simulink library "ClairvauxLibrary"  (R2020b)
settings: Solver=VariableStepAuto  StartTime=0.0  StopTime=10.0  RelTol=1e-3
undefined symbols (not defined in the file): OutMax, OutMin, Ts, w0
libraries: $bdroot x4, simulink x2, sharedtransform x2
(part 1 of 2)
settings Model: Creator=mujim  LastModifiedBy=mujim

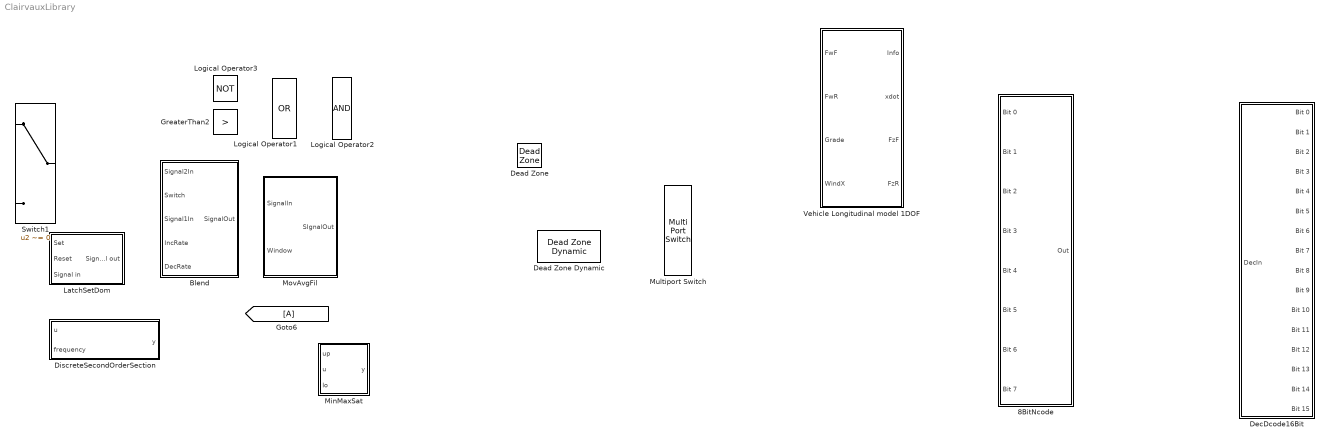
== system ClairvauxLibrary ==
  8BitNcode : Subsystem
  Blend : Subsystem
  Dead Zone : DeadZone  SaturateOnIntegerOverflow=on
  Dead Zone Dynamic : simulink/Discontinuities/Dead Zone Dynamic
      settings: SourceProductBaseCode=SL
  DecDcode16Bit : Subsystem
  DiscreteSecondOrderSection : Subsystem  mask(DiscreteSecondOrderSection){zeta=sin(1*pi/4), Ts=Ts, w0=w0}
      mask prompts: zeta "Damping ratio"; Ts "Sample time Ts"; w0 "Pre-warping frequency w0"
      mask help:
      | Implements the Tustin discretization of the second-order lowpass filter
      |
      |                          w^2
      | F(s) = ---------------------------------------
      |            s^2 + 2 * zeta * w * s + w^2
      |
      | where zeta is the damping ratio and w is the cutoff frequency value fed to the "frequency" port. The discrete transfer function is obtained by Tustin transformation with pre-warping at the frequency w0. The default value w0=0 corresponds to the usual bilinear transformation:
      |
      | s = 2/Ts (z-1)/(z+1).
      mask init:
      | if w0>0
      |    tau = tan(w0*Ts/2)/w0;
      | else
      |    tau = Ts/2;
      | end
      mask Display:
      | text(0.4,0.5,'DSOS');
      | port_label('input', 1, 'SigIn');
      | port_label('output', 1, 'SigOut');
      | port_label('input', 2, 'freq');
  GreaterThan2 : RelationalOperator  Operator=>  OutDataTypeStr=boolean  RndMeth=Zero
  LatchSetDom : Subsystem
  Logical Operator1 : Logic  Operator=OR  AllPortsSameDT=off  OutDataTypeStr=boolean
  Logical Operator2 : Logic  AllPortsSameDT=off  OutDataTypeStr=boolean
  Logical Operator3 : Logic  Operator=NOT  OutDataTypeStr=boolean
  MinMaxSat : Subsystem
  MovAvgFil : Subsystem
  Multiport Switch : MultiPortSwitch  Inputs=2  DataPortForDefault=Additional data port  DiagnosticForDefault=None  RndMeth=Zero
  Switch1 : Switch  Criteria=u2 ~= 0  OutDataTypeStr=double  RndMeth=Zero
  Vehicle Longitudinal model 1DOF : Subsystem  mask(Vehicle Longitudinal model 1DOF){NF=0, NR=0, m=0, a=0, b=0, h=0, Cd=0, Cl=0, Cpm=0, Af=0, x_o=0, xdot_o=0, Pabs=0, T=0, g=0}
      mask prompts: NF "Number of wheels on front axle, NF [-]"; NR "Number of wheels on rear axle, NR [-]"; m "Mass, m [Kg]"; a "Horizontal distance from CG to front axle, a [m]"; b "Horizontal distance from CG to rear axle, b [m]"; h "CG height above axles, h [m]"; Cd "Drag coefficient, Cd [-]"; Cl "Lift coefficient, Cl [-]"; Cpm "Pitch drag moment coeffiecient, Cpm [-]"; Af "Frontal Area, Af [m^2]"; x_o "Initial position, x_o [m]"; xdot_o "Initial velocity, xdot_o [m/s]"; Pabs "Absolute Pressure, Pabs [Pa]"; T "Air Temp, T [K]"; g "Gravitational acceleration, g [m/s^2]"
      mask DialogControl Container3 Prompt: Parameters
      mask DialogControl Container4 Prompt: Vehicle Paramters
      mask DialogControl Container11 Prompt: Environmental Parameters

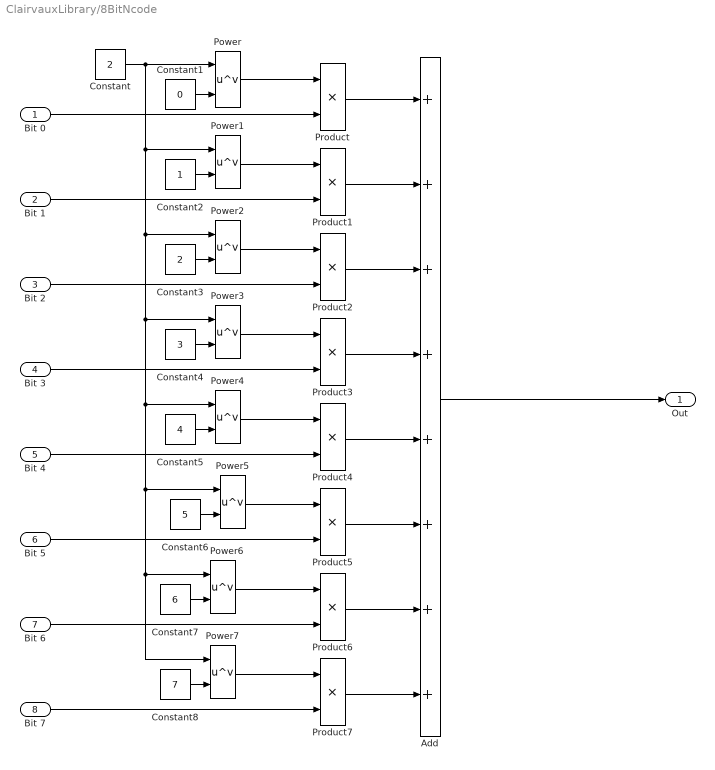
== system ClairvauxLibrary/8BitNcode ==
  Bit 0 : Inport
  Bit 1 : Inport  Port=2
  Bit 2 : Inport  Port=3
  Bit 3 : Inport  Port=4
  Bit 4 : Inport  Port=5
  Bit 5 : Inport  Port=6
  Bit 6 : Inport  Port=7
  Bit 7 : Inport  Port=8
  Add : Sum  Inputs=++++++++
  Constant : Constant  Value=2
  Constant1 : Constant  Value=0
  Constant2 : Constant
  Constant3 : Constant  Value=2
  Constant4 : Constant  Value=3
  Constant5 : Constant  Value=4
  Constant6 : Constant  Value=5
  Constant7 : Constant  Value=6
  Constant8 : Constant  Value=7
  Power{,1..7} (8 alike) : Math  Operator=pow  SaturateOnIntegerOverflow=on
  Product{,1..7} (8 alike) : Product
  Out : Outport
  wires:
  Bit 0/1 -> Product/2
  Constant/1 -> Power/1, Power1/1, Power2/1, Power3/1, Power7/1, Power6/1, Power5/1, Power4/1
  Power/1 -> Product/1
  Add/1 -> Out/1
  Constant1/1 -> Power/2
  Constant2/1 -> Power1/2
  Constant3/1 -> Power2/2
  Constant4/1 -> Power3/2
  Constant5/1 -> Power4/2
  Constant6/1 -> Power5/2
  Constant7/1 -> Power6/2
  Constant8/1 -> Power7/2
  Product/1 -> Add/1
  Product1/1 -> Add/2
  Product2/1 -> Add/3
  Product3/1 -> Add/4
  Product4/1 -> Add/5
  Product5/1 -> Add/6
  Product6/1 -> Add/7
  Product7/1 -> Add/8
  Power1/1 -> Product1/1
  Power2/1 -> Product2/1
  Power3/1 -> Product3/1
  Power4/1 -> Product4/1
  Power5/1 -> Product5/1
  Power6/1 -> Product6/1
  Power7/1 -> Product7/1
  Bit 1/1 -> Product1/2
  Bit 2/1 -> Product2/2
  Bit 3/1 -> Product3/2
  Bit 4/1 -> Product4/2
  Bit 5/1 -> Product5/2
  Bit 6/1 -> Product6/2
  Bit 7/1 -> Product7/2

== system ClairvauxLibrary/Blend ==
  note: Blend between 2 signals with a defined rate of rise and fall
      | Switch input:
      | 0 = Signal1
      | 1 = Signal2
  Signal2In : Inport
  Switch : Inport  Port=2
  Signal1In : Inport  Port=3
  IncRate : Inport  Port=4
  DecRate : Inport  Port=5
  Rate Limiter Dynamic : simulink/Discontinuities/Rate Limiter Dynamic
  Switch3 : $bdroot/Switch1  Criteria=u2 ~= 0  Threshold=0  OutMin=[]  OutMax=[]  OutDataTypeStr=double  RndMeth=Zero  SampleTime=-1  AllowDiffInputSizes=off
  SignalOut : Outport
  wires:
  Signal2In/1 -> Switch3/1
  Switch3/1 -> Rate Limiter Dynamic/2
  Rate Limiter Dynamic/1 -> SignalOut/1
  Signal1In/1 -> Switch3/3
  DecRate/1 -> Rate Limiter Dynamic/3
  Switch/1 -> Switch3/2
  IncRate/1 -> Rate Limiter Dynamic/1

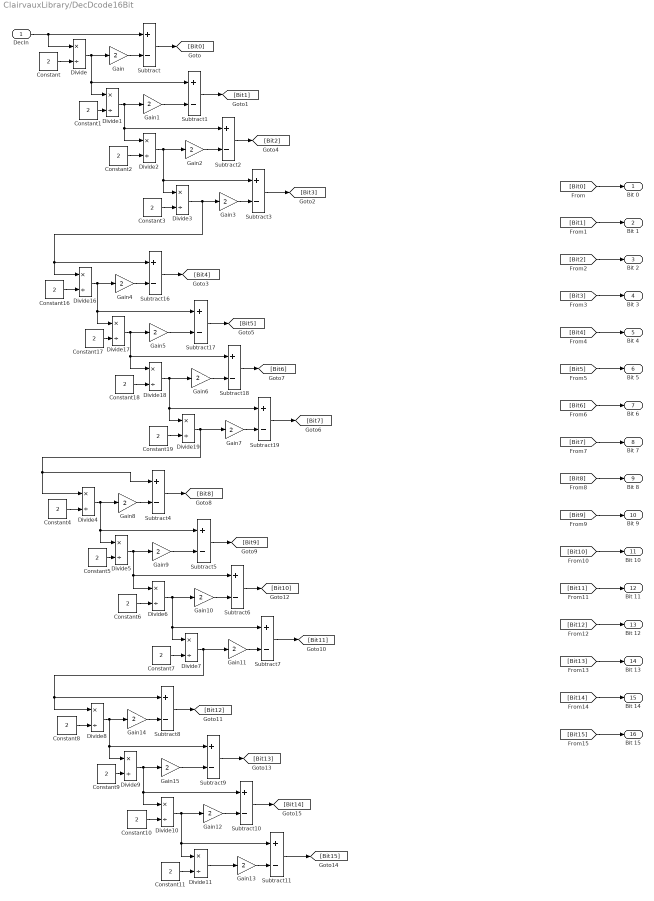
== system ClairvauxLibrary/DecDcode16Bit ==
  DecIn : Inport
  Constant{,1..11,16..19} (16 alike) : Constant  Value=2
  Divide{,1..11,16..19} (16 alike) : Product  Inputs=*/  OutDataTypeStr=fixdt('int16', 'DataTypeOverride', 'Off')
  Gain{,1..15} (16 alike) : Gain  Gain=2
  Subtract{,1..11,16..19} (16 alike) : Sum  Inputs=+-
  Bit 0 : Outport
  Bit 1 : Outport  Port=2
  Bit 2 : Outport  Port=3
  Bit 3 : Outport  Port=4
  Bit 4 : Outport  Port=5
  Bit 5 : Outport  Port=6
  Bit 6 : Outport  Port=7
  Bit 7 : Outport  Port=8
  Bit 8 : Outport  Port=9
  Bit 9 : Outport  Port=10
  Bit 10 : Outport  Port=11
  Bit 11 : Outport  Port=12
  Bit 12 : Outport  Port=13
  Bit 13 : Outport  Port=14
  Bit 14 : Outport  Port=15
  Bit 15 : Outport  Port=16
  wires:
  DecIn/1 -> Subtract/1, Divide/1
  Constant/1 -> Divide/2
  Divide/1 -> Divide1/1, Subtract1/1, Gain/1
  Divide1/1 -> Divide2/1, Subtract2/1, Gain1/1
  Constant1/1 -> Divide1/2
  Subtract/1 -> [Bit0]
  Constant2/1 -> Divide2/2
  Divide2/1 -> Divide3/1, Subtract3/1, Gain2/1
  [Bit0] -> Bit 0/1
  Subtract1/1 -> [Bit1]
  [Bit1] -> Bit 1/1
  Subtract3/1 -> [Bit3]
  Constant3/1 -> Divide3/2
  Subtract2/1 -> [Bit2]
  [Bit2] -> Bit 2/1
  [Bit3] -> Bit 3/1
  [Bit4] -> Bit 4/1
  [Bit5] -> Bit 5/1
  [Bit6] -> Bit 6/1
  [Bit7] -> Bit 7/1
  [Bit15] -> Bit 15/1
  [Bit14] -> Bit 14/1
  [Bit13] -> Bit 13/1
  [Bit12] -> Bit 12/1
  [Bit11] -> Bit 11/1
  [Bit10] -> Bit 10/1
  [Bit9] -> Bit 9/1
  [Bit8] -> Bit 8/1
  Gain/1 -> Subtract/2
  Gain1/1 -> Subtract1/2
  Gain2/1 -> Subtract2/2
  Gain3/1 -> Subtract3/2
  Gain7/1 -> Subtract19/2
  Gain6/1 -> Subtract18/2
  Gain5/1 -> Subtract17/2
  Gain4/1 -> Subtract16/2
  Divide19/1 -> Gain7/1, Subtract4/1, Divide4/1
  Subtract18/1 -> [Bit6]
  Constant19/1 -> Divide19/2
  Subtract19/1 -> [Bit7]
  Subtract17/1 -> [Bit5]
  Divide18/1 -> Gain6/1, Subtract19/1, Divide19/1
  Constant18/1 -> Divide18/2
  Subtract16/1 -> [Bit4]
  Constant17/1 -> Divide17/2
  Divide17/1 -> Gain5/1, Subtract18/1, Divide18/1
  Divide16/1 -> Gain4/1, Subtract17/1, Divide17/1
  Constant16/1 -> Divide16/2
  Divide3/1 -> Subtract16/1, Divide16/1, Gain3/1
  Constant4/1 -> Divide4/2
  Divide4/1 -> Divide5/1, Subtract5/1, Gain8/1
  Divide5/1 -> Divide6/1, Subtract6/1, Gain9/1
  Constant5/1 -> Divide5/2
  Subtract4/1 -> [Bit8]
  Constant6/1 -> Divide6/2
  Divide6/1 -> Divide7/1, Subtract7/1, Gain10/1
  Subtract5/1 -> [Bit9]
  Subtract7/1 -> [Bit11]
  Constant7/1 -> Divide7/2
  Subtract6/1 -> [Bit10]
  Divide7/1 -> Subtract8/1, Divide8/1, Gain11/1
  Gain8/1 -> Subtract4/2
  Gain9/1 -> Subtract5/2
  Gain10/1 -> Subtract6/2
  Gain11/1 -> Subtract7/2
  Gain13/1 -> Subtract11/2
  Gain12/1 -> Subtract10/2
  Gain15/1 -> Subtract9/2
  Gain14/1 -> Subtract8/2
  Divide11/1 -> Gain13/1
  Subtract10/1 -> [Bit14]
  Constant11/1 -> Divide11/2
  Subtract11/1 -> [Bit15]
  Subtract9/1 -> [Bit13]
  Divide10/1 -> Gain12/1, Subtract11/1, Divide11/1
  Constant10/1 -> Divide10/2
  Subtract8/1 -> [Bit12]
  Constant9/1 -> Divide9/2
  Divide9/1 -> Gain15/1, Subtract10/1, Divide10/1
  Divide8/1 -> Gain14/1, Subtract9/1, Divide9/1
  Constant8/1 -> Divide8/2

== system ClairvauxLibrary/DiscreteSecondOrderSection ==
  u : Inport
  frequency : Inport  Port=2
  Constant : Constant  Value=zeta
  Constant1 : Constant  Value=tau
  Gain1 : Gain  Gain=2
  MATLAB Function : MATLAB Function  Tag=#GainSurfaceTarget_  TreatAsAtomicUnit=on
  Product1 : Product
  Product2 : Product
  Product5 : Product
  Sum : Sum  Inputs=|++
  Sum1 : Sum  Inputs=++|
  Sum2 : Sum  Inputs=+|+
  Sum3 : Sum  Inputs=+|-
  Unit Delay1 : UnitDelay  SampleTime=Ts  HasFrameUpgradeWarning=on
  Unit Delay2 : UnitDelay  SampleTime=Ts  HasFrameUpgradeWarning=on
  y : Outport  VectorParamsAs1DForOutWhenUnconnected=off
  wires:
  Unit Delay1/1 -> Sum/2
  MATLAB Function/3(c) -> Product2/2
  MATLAB Function/2(b) -> Product5/2
  Product2/1 -> Sum3/2
  Constant1/1 -> MATLAB Function/3(tau)
  MATLAB Function/1(a) -> Product1/2
  frequency/1 -> MATLAB Function/1(w)
  Sum1/1 -> Unit Delay1/1
  Sum3/1 -> Unit Delay2/1
  Sum2/1 -> Gain1/1
  Constant/1 -> MATLAB Function/2(zeta)
  Product1/1 -> y/1
  u/1 -> Sum3/1, Sum2/1, Sum/1
  Unit Delay2/1 -> Sum1/2
  Sum/1 -> Product1/1, Product5/1, Product2/1
  Product5/1 -> Sum2/2
  Gain1/1 -> Sum1/1

== system ClairvauxLibrary/LatchSetDom ==
  Set : Inport
  Reset : Inport  Port=2
  Signal in : Inport  Port=3
  Signal out : Outport

== system ClairvauxLibrary/MinMaxSat ==
  up : Inport
  u : Inport  Port=2
  lo : Inport  Port=3
  LowerRelop1 : RelationalOperator  DisableCoverage=on  Operator=>  OutDataTypeStr=boolean  RndMeth=Nearest
  Switch : Switch  Criteria=u2 ~= 0  OutDataTypeStr=Inherit: Inherit via back propagation  ZeroCross=off
  Switch2 : Switch  Criteria=u2 ~= 0  OutMin=OutMin  OutMax=OutMax  OutDataTypeStr=Inherit: Inherit via back propagation  ZeroCross=off
  UpperRelop : RelationalOperator  DisableCoverage=on  Operator=<  OutDataTypeStr=boolean  RndMeth=Nearest
  y : Outport  OutMin=OutMin  OutMax=OutMax
  wires:
  Switch/1 -> Switch2/3
  LowerRelop1/1 -> Switch2/2
  UpperRelop/1 -> Switch/2
  Switch2/1 -> y/1
  u/1 -> LowerRelop1/1, Switch/3, UpperRelop/1
  up/1 -> Switch2/1, LowerRelop1/2
  lo/1 -> Switch/1, UpperRelop/2

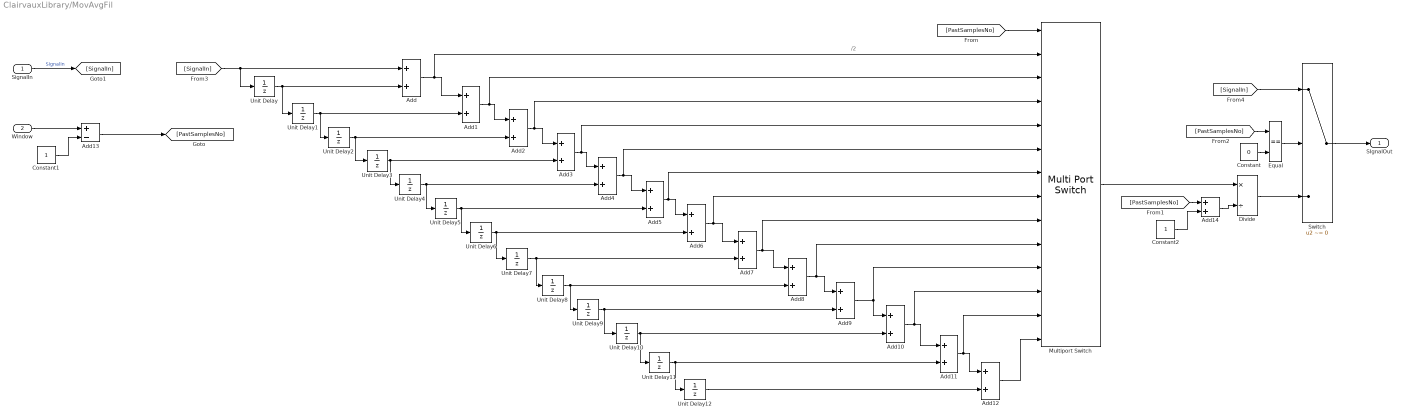
== system ClairvauxLibrary/MovAvgFil ==
  note: /2
  SignalIn : Inport
  Window : Inport  Port=2
  Add{,1..12,14} (14 alike) : Sum
  Add13 : Sum  Inputs=+-
  Constant : Constant  Value=0
  Constant1 : Constant
  Constant2 : Constant
  Divide : Product  Inputs=*/
  Equal : RelationalOperator  Operator===  OutDataTypeStr=boolean  RndMeth=Simplest
  Multiport Switch : MultiPortSwitch  Inputs=13
  Switch : Switch  Criteria=u2 ~= 0  RndMeth=Zero
  Unit Delay{,1..12} (13 alike) : UnitDelay  SampleTime=-1  HasFrameUpgradeWarning=on
  SIgnalOut : Outport
  wires:
  Divide/1 -> Switch/3
  [SignalIn] -> Switch/1
  Switch/1 -> SIgnalOut/1
  Equal/1 -> Switch/2
  [SignalIn] -> Unit Delay/1, Add/1
  Constant/1 -> Equal/2
  [PastSamplesNo] -> Equal/1
  [PastSamplesNo] -> Multiport Switch/1
  Multiport Switch/1 -> Divide/1
  Add12/1 -> Multiport Switch/14
  Add11/1 -> Multiport Switch/13, Add12/1
  Add10/1 -> Multiport Switch/12, Add11/1
  Unit Delay11/1 -> Unit Delay12/1, Add11/2
  Add9/1 -> Add10/1, Multiport Switch/11
  Add8/1 -> Multiport Switch/10, Add9/1
  Add7/1 -> Multiport Switch/9, Add8/1
  Add6/1 -> Multiport Switch/8, Add7/1
  Add5/1 -> Multiport Switch/7, Add6/1
  Add4/1 -> Multiport Switch/6, Add5/1
  Add3/1 -> Multiport Switch/5, Add4/1
  Add2/1 -> Multiport Switch/4, Add3/1
  Add1/1 -> Multiport Switch/3, Add2/1
  Add/1 -> Multiport Switch/2, Add1/1
  Unit Delay4/1 -> Unit Delay5/1, Add4/2
  Unit Delay2/1 -> Unit Delay3/1, Add2/2
  Unit Delay7/1 -> Add7/2, Unit Delay8/1
  Unit Delay8/1 -> Unit Delay9/1, Add8/2
  Unit Delay3/1 -> Unit Delay4/1, Add3/2
  Unit Delay12/1 -> Add12/2
  Unit Delay6/1 -> Add6/2, Unit Delay7/1
  SignalIn/1 -> [SignalIn]  "SignalIn"
  Unit Delay10/1 -> Unit Delay11/1, Add10/2
  Unit Delay1/1 -> Unit Delay2/1, Add1/2
  Unit Delay/1 -> Unit Delay1/1, Add/2
  Unit Delay9/1 -> Unit Delay10/1, Add9/2
  Unit Delay5/1 -> Add5/2, Unit Delay6/1
  Add13/1 -> [PastSamplesNo]
  Window/1 -> Add13/1
  Constant1/1 -> Add13/2
  Constant2/1 -> Add14/2
  [PastSamplesNo] -> Add14/1
  Add14/1 -> Divide/2

== system ClairvauxLibrary/Vehicle Longitudinal model 1DOF ==
  FwF : Inport
  FwR : Inport  Port=2
  Grade : Inport  Port=3
  WindX : Inport  Port=4
  AirTempConstant : Constant  Value=T
  FExtConstant : Constant  Value=[0,0,0]
  MExtConstant : Constant  Value=[0,0,0]
  Subsystem : Subsystem
  Info : Outport  VectorParamsAs1DForOutWhenUnconnected=off
  xdot : Outport  Port=2  PortDimensions=1  VectorParamsAs1DForOutWhenUnconnected=off
  FzF : Outport  Port=3  PortDimensions=1  VectorParamsAs1DForOutWhenUnconnected=off
  FzR : Outport  Port=4  PortDimensions=1  VectorParamsAs1DForOutWhenUnconnected=off
  wires:
  Subsystem/4(FzR) -> FzR/1
  FwF/1 -> Subsystem/1(FwF)
  FwR/1 -> Subsystem/2(FwR)
  Subsystem/1(Info) -> Info/1
  AirTempConstant/1 -> Subsystem/7(Temp)
  WindX/1 -> Subsystem/4(wind)
  MExtConstant/1 -> Subsystem/6(MExt)
  Subsystem/3(FzF) -> FzF/1
  FExtConstant/1 -> Subsystem/5(FExt)
  Grade/1 -> Subsystem/3(Grade)
  Subsystem/2(xdot) -> xdot/1

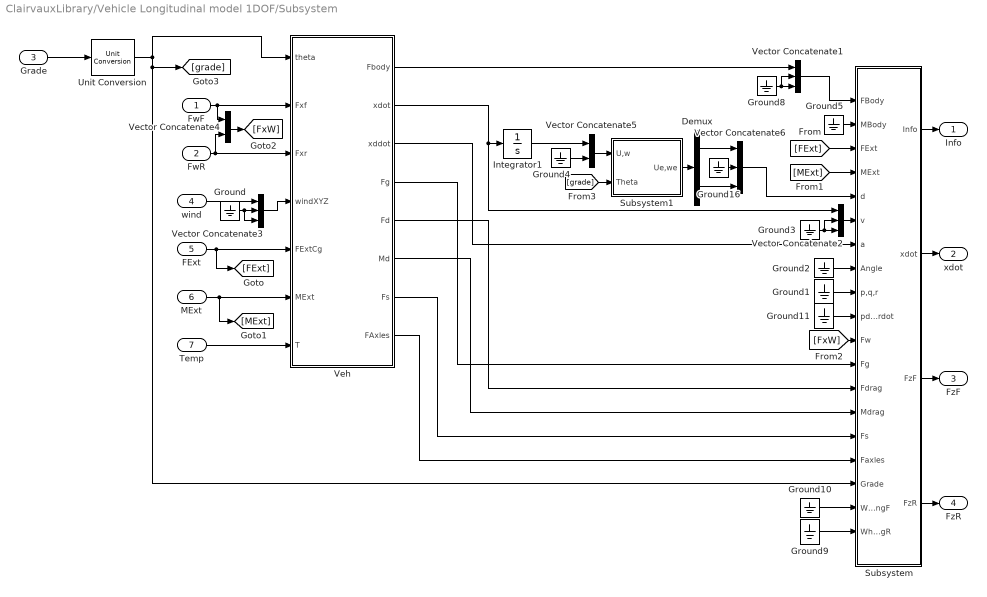
== system ClairvauxLibrary/Vehicle Longitudinal model 1DOF/Subsystem ==
  FwF : Inport  Unit=N
  FwR : Inport  Port=2  Unit=N
  Grade : Inport  Port=3  Unit=deg
  wind : Inport  Port=4  Unit=m/s
  FExt : Inport  Port=5  Unit=N
  MExt : Inport  Port=6  Unit=N*m
  Temp : Inport  Port=7  OutMin=eps  Unit=K
  Demux : Demux  Outputs=2
  Ground{,1..5,8..11,16} (11 alike) : Ground
  Integrator1 : Integrator  InitialCondition=x_o
  Subsystem : Subsystem
  Subsystem1 : Subsystem
  Unit Conversion : UnitConversion
  Vector Concatenate{1..3,6} (4 alike) : Concatenate  NumInputs=3
  Vector Concatenate4 : Concatenate
  Vector Concatenate5 : Concatenate
  Veh : Subsystem
  Info : Outport  VectorParamsAs1DForOutWhenUnconnected=off
  xdot : Outport  Port=2  Unit=m/s  VectorParamsAs1DForOutWhenUnconnected=off
  FzF : Outport  Port=3  Unit=N  VectorParamsAs1DForOutWhenUnconnected=off
  FzR : Outport  Port=4  Unit=N  VectorParamsAs1DForOutWhenUnconnected=off
  wires:
  MExt/1 -> Veh/6(MExt), [MExt]
  [MExt] -> Subsystem/4(MExt)
  Veh/7(Fs) -> Subsystem/15(Fs)
  Ground9/1 -> Subsystem/19(WhlAngR)
  Vector Concatenate5/1 -> Subsystem1/1(U,w)
  Ground4/1 -> Vector Concatenate5/2
  Ground16/1 -> Vector Concatenate6/2
  Veh/4(Fg) -> Subsystem/12(Fg)
  Demux/1 -> Vector Concatenate6/1
  Subsystem1/1(Ue,we) -> Demux/1
  Vector Concatenate3/1 -> Veh/4(windXYZ)
  Veh/5(Fd) -> Subsystem/13(Fdrag)
  Unit Conversion/1 -> Veh/1(theta), Subsystem/17(Grade), [grade]
  Ground5/1 -> Subsystem/2(MBody)
  [FxW] -> Subsystem/11(Fw)
  Ground11/1 -> Subsystem/10(pdot,qdot,rdot)
  Vector Concatenate2/1 -> Subsystem/6(v)
  Veh/3(xddot) -> Subsystem/7(a)
  Veh/6(Md) -> Subsystem/14(Mdrag)
  Demux/2 -> Vector Concatenate6/3
  FwF/1 -> Veh/2(Fxf), Vector Concatenate4/1
  Ground1/1 -> Subsystem/9(p,q,r)
  Subsystem/1(Info) -> Info/1
  Ground10/1 -> Subsystem/18(WhlAngF)
  FwR/1 -> Veh/3(Fxr), Vector Concatenate4/2
  Subsystem/4(FzR) -> FzR/1
  Vector Concatenate4/1 -> [FxW]
  Veh/8(FAxles) -> Subsystem/16(Faxles)
  Veh/2(xdot) -> Integrator1/1, Vector Concatenate2/1
  Ground3/1 -> Vector Concatenate2/3, Vector Concatenate2/2
  Grade/1 -> Unit Conversion/1
  Subsystem/2(xdot) -> xdot/1
  Subsystem/3(FzF) -> FzF/1
  Ground2/1 -> Subsystem/8(Angle)
  Integrator1/1 -> Vector Concatenate5/1
  [FExt] -> Subsystem/3(FExt)
  Vector Concatenate1/1 -> Subsystem/1(FBody)
  FExt/1 -> Veh/5(FExtCg), [FExt]
  Veh/1(Fbody) -> Vector Concatenate1/1
  Temp/1 -> Veh/7(T)
  Vector Concatenate6/1 -> Subsystem/5(d)
  [grade] -> Subsystem1/2(Theta)
  Ground8/1 -> Vector Concatenate1/2, Vector Concatenate1/3
  wind/1 -> Vector Concatenate3/1
  Ground/1 -> Vector Concatenate3/3, Vector Concatenate3/2

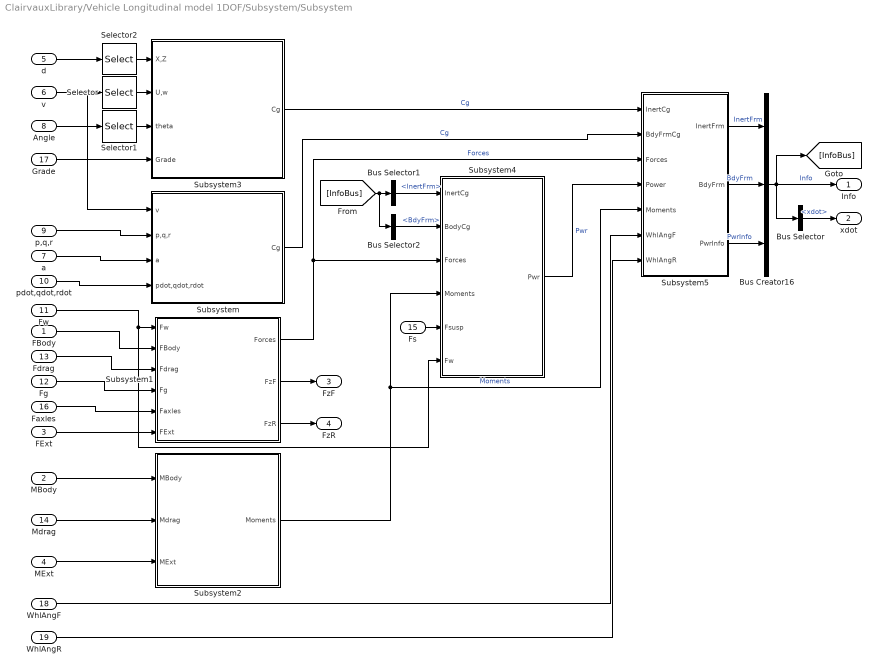
== system ClairvauxLibrary/Vehicle Longitudinal model 1DOF/Subsystem/Subsystem ==
  FBody : Inport
  MBody : Inport  Port=2  Unit=N*m
  FExt : Inport  Port=3  Unit=N
  MExt : Inport  Port=4  Unit=N*m
  d : Inport  Port=5  Unit=m
  v : Inport  Port=6  Unit=m/s
  a : Inport  Port=7  Unit=m/s^2
  Angle : Inport  Port=8  Unit=rad
  p,q,r : Inport  Port=9  Unit=rad/s
  pdot,qdot,rdot : Inport  Port=10  Unit=rad/s^2
  Fw : Inport  Port=11
  Fg : Inport  Port=12  Unit=N
  Fdrag : Inport  Port=13  Unit=N
  Mdrag : Inport  Port=14  Unit=N*m
  Fs : Inport  Port=15  Unit=N
  Faxles : Inport  Port=16  Unit=N
  Grade : Inport  Port=17  Unit=rad
  WhlAngF : Inport  Port=18  Unit=rad
  WhlAngR : Inport  Port=19  Unit=rad
  Bus Creator16 : BusCreator  Inputs=3
  Bus Selector : BusSelector  OutputSignals=BdyFrm.Cg.Vel.xdot
  Bus Selector1 : BusSelector  OutputSignals=InertFrm
  Bus Selector2 : BusSelector  OutputSignals=BdyFrm
  Selector : Selector  InputPortWidth=3  IndexOptions=Index vector (dialog)  Indices=[1 3]  OutputSizes=1
  Selector1 : Selector  InputPortWidth=3  IndexOptions=Index vector (dialog)  Indices=[2]  OutputSizes=1
  Selector2 : Selector  InputPortWidth=3  IndexOptions=Index vector (dialog)  Indices=[1 3]  OutputSizes=1
  Subsystem : Subsystem
  Subsystem1 : Subsystem
  Subsystem2 : Subsystem
  Subsystem3 : Subsystem
  Subsystem4 : Subsystem
  Subsystem5 : Subsystem
  Info : Outport  VectorParamsAs1DForOutWhenUnconnected=off
  xdot : Outport  Port=2  VectorParamsAs1DForOutWhenUnconnected=off
  FzF : Outport  Port=3  VectorParamsAs1DForOutWhenUnconnected=off
  FzR : Outport  Port=4  VectorParamsAs1DForOutWhenUnconnected=off
  wires:
  Bus Selector/1 -> xdot/1  "<xdot>"
  Fg/1 -> Subsystem1/4(Fg)
  Subsystem/1(Cg) -> Subsystem5/2(BdyFrmCg)  "Cg"
  Grade/1 -> Subsystem3/4(Grade)
  Subsystem2/1(Moments) -> Subsystem5/5(Moments), Subsystem4/4(Moments)  "Moments"
  Subsystem1/3(FzR) -> FzR/1
  Bus Creator16/1 -> [InfoBus], Bus Selector/1, Info/1  "Info"
  MBody/1 -> Subsystem2/1(MBody)
  Selector1/1 -> Subsystem3/3(theta)
  Fw/1 -> Subsystem1/1(Fw), Subsystem4/6(Fw)
  Subsystem1/1(Forces) -> Subsystem5/3(Forces), Subsystem4/3(Forces)  "Forces"
  a/1 -> Subsystem/3(a)
  Fs/1 -> Subsystem4/5(Fsusp)
  MExt/1 -> Subsystem2/3(MExt)
  Mdrag/1 -> Subsystem2/2(Mdrag)
  Selector/1 -> Subsystem3/2(U,w)
  Bus Selector2/1 -> Subsystem4/2(BodyCg)  "<BdyFrm>"
  Selector2/1 -> Subsystem3/1(X,Z)
  Subsystem4/1(Pwr) -> Subsystem5/4(Power)  "Pwr"
  Subsystem5/1(InertFrm) -> Bus Creator16/1  "InertFrm"
  WhlAngR/1 -> Subsystem5/7(WhlAngR)
  d/1 -> Selector2/1
  Angle/1 -> Selector1/1
  Bus Selector1/1 -> Subsystem4/1(InertCg)  "<InertFrm>"
  pdot,qdot,rdot/1 -> Subsystem/4(pdot,qdot,rdot)
  [InfoBus] -> Bus Selector2/1, Bus Selector1/1
  p,q,r/1 -> Subsystem/2(p,q,r)
  Subsystem5/3(PwrInfo) -> Bus Creator16/3  "PwrInfo"
  v/1 -> Subsystem/1(v), Selector/1
  WhlAngF/1 -> Subsystem5/6(WhlAngF)
  FBody/1 -> Subsystem1/2(FBody)
  Fdrag/1 -> Subsystem1/3(Fdrag)
  Subsystem3/1(Cg) -> Subsystem5/1(InertCg)  "Cg"
  Faxles/1 -> Subsystem1/5(Faxles)
  FExt/1 -> Subsystem1/6(FExt)
  Subsystem5/2(BdyFrm) -> Bus Creator16/2  "BdyFrm"
  Subsystem1/2(FzF) -> FzF/1

== system ClairvauxLibrary/Vehicle Longitudinal model 1DOF/Subsystem/Subsystem1 ==
  U,w : Inport
  Theta : Inport  Port=2
  Constant : Constant  Value=0
  Mux3 : Mux  Inputs=3
  Mux4 : Mux  Inputs=3
  Product : Product  Multiplication=Matrix(*)  SaturateOnIntegerOverflow=on  OutDataTypeStr=Inherit: Same as first input
  Rotation Angles to Direction Cosine Matrix : sharedtransform/Rotation Angles to Direction Cosine Matrix  rotationOrder=ZYX  aMode=aMode
      settings: SourceProductBaseCode=AE,PW,MT,UV,VE,VP
  Selector : Selector  InputPortWidth=2  IndexOptions=Index vector (dialog)  Indices=1  OutputSizes=1
  Selector1 : Selector  InputPortWidth=3  IndexOptions=Index vector (dialog)  Indices=[1 3]  OutputSizes=1
  Selector2 : Selector  InputPortWidth=2  IndexOptions=Index vector (dialog)  Indices=2  OutputSizes=1
  Transpose : Math  Operator=transpose  SignedPower=on  SaturateOnIntegerOverflow=on
  Ue,we : Outport  Unit=m/s  VectorParamsAs1DForOutWhenUnconnected=off
  wires:
  U,w/1 -> Selector/1, Selector2/1
  Selector2/1 -> Mux4/3
  Rotation Angles to Direction Cosine Matrix/1 -> Transpose/1
  Constant/1 -> Mux3/1, Mux4/2, Mux3/3
  Mux3/1 -> Rotation Angles to Direction Cosine Matrix/1
  Selector1/1 -> Ue,we/1
  Product/1 -> Selector1/1
  Selector/1 -> Mux4/1
  Theta/1 -> Mux3/2
  Transpose/1 -> Product/1
  Mux4/1 -> Product/2

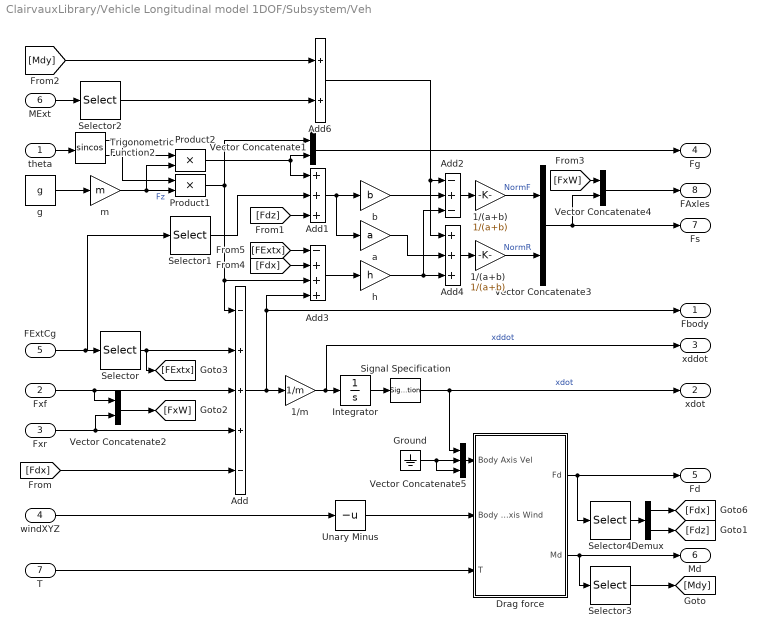
== system ClairvauxLibrary/Vehicle Longitudinal model 1DOF/Subsystem/Veh ==
  theta : Inport  Unit=rad
  Fxf : Inport  Port=2
  Fxr : Inport  Port=3
  windXYZ : Inport  Port=4
  FExtCg : Inport  Port=5
  MExt : Inport  Port=6
  T : Inport  Port=7
  1/(a+b) : Gain  Gain=1/(a+b)
  "1/(a+b) " : Gain  Gain=1/(a+b)
  1/m : Gain  Gain=1/m
  Add : Sum  Inputs=-+++-
  Add1 : Sum  Inputs=+++
  Add2 : Sum  Inputs=-+-
  Add3 : Sum  Inputs=-+++
  Add4 : Sum  Inputs=+++
  Add6 : Sum
  Demux : Demux  Outputs=2
  Drag force : Subsystem  mask{A=Af, beta_w=[-1,1], Cd=Cd, Cs=[0,0], Cl=Cl, Cpm=Cpm, Lcpm=a+b, Crm=[0,0], Cym=[0,0], R=287.058, Pabs=Pabs}
      mask prompts: A "Effective area, A [m^s2]:"; beta_w "Relative wind angle vector, beta_w [rad]:"; Cd "Longitudinal drag coefficient, Cd [-]:"; Cs "Side force coefficient data, Cs [-]:"; Cl "Lift coefficient, Cl [-]:"; Cpm "Pitch moment coefficient, Cpm [-]:"; Lcpm "Pitch moment length, Lcpm"; Crm "Roll moment coefficient data, Crm [-]:"; Cym "Yaw moment coefficient data, Cym [-]:"; R "Gas constant, R [J/(kg*K)]:"; Pabs "Absoulte pressure, Pabs [Pa]:"
  Ground : Ground
  Integrator : Integrator  InitialCondition=xdot_o
  Product1 : Product
  Product2 : Product
  Selector : Selector  InputPortWidth=3  IndexOptions=Index vector (dialog)  Indices=[1]  OutputSizes=1
  Selector1 : Selector  InputPortWidth=3  IndexOptions=Index vector (dialog)  Indices=[3]  OutputSizes=1
  Selector2 : Selector  InputPortWidth=3  IndexOptions=Index vector (dialog)  Indices=[2]  OutputSizes=1
  Selector3 : Selector  InputPortWidth=3  IndexOptions=Index vector (dialog)  Indices=[2]  OutputSizes=1
  Selector4 : Selector  InputPortWidth=3  IndexOptions=Index vector (dialog)  Indices=[1 3]  OutputSizes=1
  Signal Specification : SignalSpecification  Unit=m/s  Dimensions=1
  Trigonometric Function2 : Trigonometry  Operator=sincos
  Unary Minus : UnaryMinus
  Vector Concatenate1 : Concatenate
  Vector Concatenate2 : Concatenate
  Vector Concatenate3 : Concatenate
  Vector Concatenate4 : Concatenate  Mode=Multidimensional array  ConcatenateDimension=2
  Vector Concatenate5 : Concatenate  NumInputs=3
  a : Gain  Gain=a
  b : Gain  Gain=b
  g : Constant  Value=g
  h : Gain  Gain=h
  m : Gain  Gain=m
  Fbody : Outport  VectorParamsAs1DForOutWhenUnconnected=off
  xdot : Outport  Port=2  VectorParamsAs1DForOutWhenUnconnected=off
  xddot : Outport  Port=3  VectorParamsAs1DForOutWhenUnconnected=off
  Fg : Outport  Port=4  VectorParamsAs1DForOutWhenUnconnected=off
  Fd : Outport  Port=5  VectorParamsAs1DForOutWhenUnconnected=off
  Md : Outport  Port=6  VectorParamsAs1DForOutWhenUnconnected=off
  Fs : Outport  Port=7  VectorParamsAs1DForOutWhenUnconnected=off
  FAxles : Outport  Port=8  VectorParamsAs1DForOutWhenUnconnected=off
  wires:
  FExtCg/1 -> Selector/1, Selector1/1
  1/(a+b)/1 -> Vector Concatenate3/1  "NormF"
  Fxf/1 -> Vector Concatenate2/1, Add/3
  Add/1 -> 1/m/1, Fbody/1, Add3/4
  Unary Minus/1 -> Drag force/2(Body Axis Wind)
  Vector Concatenate2/1 -> [FxW]
  Ground/1 -> Vector Concatenate5/2, Vector Concatenate5/3
  Product2/1 -> Add1/1, Vector Concatenate1/2
  Selector/1 -> Add/2, [FExtx]
  Trigonometric Function2/2 -> Product2/1
  Add2/1 -> 1/(a+b)/1
  Vector Concatenate5/1 -> Drag force/1(Body Axis Vel)
  Vector Concatenate1/1 -> Fg/1
  Selector4/1 -> Demux/1
  b/1 -> Add2/2
  1/m/1 -> Integrator/1, xddot/1  "xddot"
  Add1/1 -> b/1, a/1
  Integrator/1 -> Signal Specification/1
  Demux/2 -> [Fdz]
  Vector Concatenate3/1 -> Fs/1, Vector Concatenate4/2
  T/1 -> Drag force/3(T)
  theta/1 -> Trigonometric Function2/1
  [Fdx] -> Add3/2
  Selector2/1 -> Add6/2
  m/1 -> Product1/2, Product2/2  "Fz"
  Selector1/1 -> Add1/2
  h/1 -> Add4/3, Add2/3
  MExt/1 -> Selector2/1
  [FxW] -> Vector Concatenate4/1
  Add4/1 -> "1/(a+b) "/1
  Vector Concatenate4/1 -> FAxles/1
  [Fdx] -> Add/5
  Add6/1 -> Add2/1, Add4/1
  Drag force/1(Fd) -> Fd/1, Selector4/1
  Drag force/2(Md) -> Md/1, Selector3/1
  Trigonometric Function2/1 -> Product1/1
  "1/(a+b) "/1 -> Vector Concatenate3/2  "NormR"
  Fxr/1 -> Vector Concatenate2/2, Add/4
  Selector3/1 -> [Mdy]
  Demux/1 -> [Fdx]
  [Fdz] -> Add1/3
  windXYZ/1 -> Unary Minus/1
  [Mdy] -> Add6/1
  Product1/1 -> Add3/3, Add/1, Vector Concatenate1/1
  a/1 -> Add4/2
  Add3/1 -> h/1
  Signal Specification/1 -> Vector Concatenate5/1, xdot/1  "xdot"
  g/1 -> m/1
  [FExtx] -> Add3/1

== system ClairvauxLibrary/Vehicle Longitudinal model 1DOF/Subsystem/Subsystem/Subsystem ==
  v : Inport  Unit=m/s
  p,q,r : Inport  Port=2  Unit=rad/s
  a : Inport  Port=3  Unit=m/s^2
  pdot,qdot,rdot : Inport  Port=4
  Subsystem : Subsystem
  Cg : Outport  VectorParamsAs1DForOutWhenUnconnected=off
  wires:
  Subsystem/1(Cg) -> Cg/1
  v/1 -> Subsystem/1(v)
  p,q,r/1 -> Subsystem/2(p,q,r)
  a/1 -> Subsystem/3(a)
  pdot,qdot,rdot/1 -> Subsystem/4(pdot,qdot,rdot)

== system ClairvauxLibrary/Vehicle Longitudinal model 1DOF/Subsystem/Subsystem/Subsystem1 ==
  Fw : Inport
  FBody : Inport  Port=2
  Fdrag : Inport  Port=3
  Fg : Inport  Port=4
  Faxles : Inport  Port=5
  FExt : Inport  Port=6
  Subsystem : Subsystem
  Terminator : Terminator
  Forces : Outport  VectorParamsAs1DForOutWhenUnconnected=off
  FzF : Outport  Port=2  VectorParamsAs1DForOutWhenUnconnected=off
  FzR : Outport  Port=3  VectorParamsAs1DForOutWhenUnconnected=off
  wires:
  Fdrag/1 -> Subsystem/1(Fdrag)
  FBody/1 -> Subsystem/5(FBody)
  Fg/1 -> Subsystem/2(Fg)
  Faxles/1 -> Subsystem/3(Faxles)
  FExt/1 -> Subsystem/4(FExt)
  Subsystem/3(FzR) -> FzR/1
  Subsystem/2(FzF) -> FzF/1
  Subsystem/1(Forces) -> Forces/1
  Fw/1 -> Terminator/1

== system ClairvauxLibrary/Vehicle Longitudinal model 1DOF/Subsystem/Subsystem/Subsystem2 ==
  MBody : Inport
  Mdrag : Inport  Port=2  PortDimensions=3
  MExt : Inport  Port=3  PortDimensions=3
  Bus Creator{1,3,7,24} (4 alike) : BusCreator  Inputs=3
  Demux : Demux  Outputs=3
  Demux1 : Demux  Outputs=3
  Demux2 : Demux  Outputs=3
  Signal Specification{1..8,23} (9 alike) : SignalSpecification  Unit=N*m
  Moments : Outport  VectorParamsAs1DForOutWhenUnconnected=off
  wires:
  Signal Specification2/1 -> Bus Creator24/3  "Mz"
  Signal Specification8/1 -> Bus Creator3/1  "Mx"
  Signal Specification6/1 -> Bus Creator3/2  "My"
  Signal Specification4/1 -> Bus Creator1/3  "Mz"
  Bus Creator1/1 -> Bus Creator7/2  "Drag"
  Signal Specification5/1 -> Bus Creator1/1  "Mx"
  Demux1/1 -> Signal Specification5/1
  Demux1/3 -> Signal Specification4/1
  Signal Specification7/1 -> Bus Creator3/3  "Mz"
  Bus Creator7/1 -> Moments/1  "Moments"
  Signal Specification3/1 -> Bus Creator1/2  "My"
  MBody/1 -> Demux/1
  Demux1/2 -> Signal Specification3/1
  Mdrag/1 -> Demux1/1
  Demux/3 -> Signal Specification2/1
  MExt/1 -> Demux2/1
  Demux/1 -> Signal Specification23/1
  Signal Specification23/1 -> Bus Creator24/1  "Mx"
  Signal Specification1/1 -> Bus Creator24/2  "My"
  Demux2/3 -> Signal Specification7/1
  Bus Creator3/1 -> Bus Creator7/3  "Ext"
  Demux/2 -> Signal Specification1/1
  Demux2/1 -> Signal Specification8/1
  Bus Creator24/1 -> Bus Creator7/1  "Body"
  Demux2/2 -> Signal Specification6/1

== system ClairvauxLibrary/Vehicle Longitudinal model 1DOF/Subsystem/Subsystem/Subsystem3 ==
  X,Z : Inport  Unit=m
  U,w : Inport  Port=2
  theta : Inport  Port=3
  Grade : Inport  Port=4
  Add : Sum
  Bus Creator{6..7,11,24} (4 alike) : BusCreator  Inputs=3
  Constant{1..2,10,12} (4 alike) : Constant  Value=0
  Demux : Demux  Outputs=2
  Demux5 : Demux  Outputs=2
  Signal Specification1 : SignalSpecification  Unit=rad
  Signal Specification2 : SignalSpecification  Unit=rad
  Signal Specification23 : SignalSpecification  Unit=m
  Signal Specification24 : SignalSpecification  Unit=m
  Signal Specification25 : SignalSpecification  Unit=m
  Signal Specification26 : SignalSpecification  Unit=rad
  Signal Specification7 : SignalSpecification  Unit=m/s
  Signal Specification8 : SignalSpecification  Unit=m/s
  Signal Specification9 : SignalSpecification  Unit=m/s
  Subsystem : Subsystem
  Cg : Outport  VectorParamsAs1DForOutWhenUnconnected=off
  wires:
  X,Z/1 -> Demux5/1  "XZ"
  Signal Specification1/1 -> Bus Creator11/1  "phi"
  Grade/1 -> Add/1
  Signal Specification26/1 -> Bus Creator11/2  "theta"
  theta/1 -> Signal Specification26/1, Add/2
  Constant1/1 -> Signal Specification1/1
  Constant12/1 -> Signal Specification24/1  "Y"
  Constant2/1 -> Signal Specification2/1
  U,w/1 -> Subsystem/1(U,w)
  Demux/2 -> Signal Specification9/1  "Zdot"
  Bus Creator7/1 -> Cg/1  "Cg"
  Add/1 -> Subsystem/2(Theta)
  Bus Creator11/1 -> Bus Creator7/3  "Ang"
  Subsystem/1(Ue,we) -> Demux/1
  Signal Specification7/1 -> Bus Creator6/2  "Ydot"
  Constant10/1 -> Signal Specification7/1
  Signal Specification23/1 -> Bus Creator24/1  "X"
  Bus Creator24/1 -> Bus Creator7/1  "Disp"
  Signal Specification8/1 -> Bus Creator6/1  "Xdot"
  Demux/1 -> Signal Specification8/1  "Xdot"
  Signal Specification25/1 -> Bus Creator24/3  "Z"
  Bus Creator6/1 -> Bus Creator7/2  "Vel"
  Signal Specification9/1 -> Bus Creator6/3  "Zdot"
  Demux5/1 -> Signal Specification23/1  "X"
  Demux5/2 -> Signal Specification25/1  "Z"
  Signal Specification24/1 -> Bus Creator24/2  "Y"
  Signal Specification2/1 -> Bus Creator11/3  "psi"

== system ClairvauxLibrary/Vehicle Longitudinal model 1DOF/Subsystem/Subsystem/Subsystem4 ==
  InertCg : Inport
  BodyCg : Inport  Port=2
  Forces : Inport  Port=3
  Moments : Inport  Port=4
  Fsusp : Inport  Port=5
  Fw : Inport  Port=6
  Subsystem : Subsystem
  Terminator : Terminator
  Terminator1 : Terminator
  Pwr : Outport  VectorParamsAs1DForOutWhenUnconnected=off
  wires:
  Fw/1 -> Terminator1/1
  Fsusp/1 -> Terminator/1
  InertCg/1 -> Subsystem/1(InertCg)
  BodyCg/1 -> Subsystem/2(BodyCg)
  Forces/1 -> Subsystem/3(Forces)
  Moments/1 -> Subsystem/4(Moments)
  Subsystem/1(Pwr) -> Pwr/1

== system ClairvauxLibrary/Vehicle Longitudinal model 1DOF/Subsystem/Subsystem/Subsystem5 ==
  InertCg : Inport
  BdyFrmCg : Inport  Port=2
  Forces : Inport  Port=3
  Power : Inport  Port=4
  Moments : Inport  Port=5
  WhlAngF : Inport  Port=6
  WhlAngR : Inport  Port=7
  Subsystem : Subsystem
  InertFrm : Outport  VectorParamsAs1DForOutWhenUnconnected=off
  BdyFrm : Outport  Port=2  VectorParamsAs1DForOutWhenUnconnected=off
  PwrInfo : Outport  Port=3  VectorParamsAs1DForOutWhenUnconnected=off
  wires:
  InertCg/1 -> Subsystem/1(InertCg)
  Subsystem/1(InertFrm) -> InertFrm/1
  Subsystem/2(BdyFrm) -> BdyFrm/1
  Subsystem/3(PwrInfo) -> PwrInfo/1
  BdyFrmCg/1 -> Subsystem/2(BdyFrmCg)
  Forces/1 -> Subsystem/3(Forces)
  Power/1 -> Subsystem/4(Power)
  Moments/1 -> Subsystem/5(Moments)
  WhlAngF/1 -> Subsystem/6(WhlAngF)
  WhlAngR/1 -> Subsystem/7(WhlAngR)

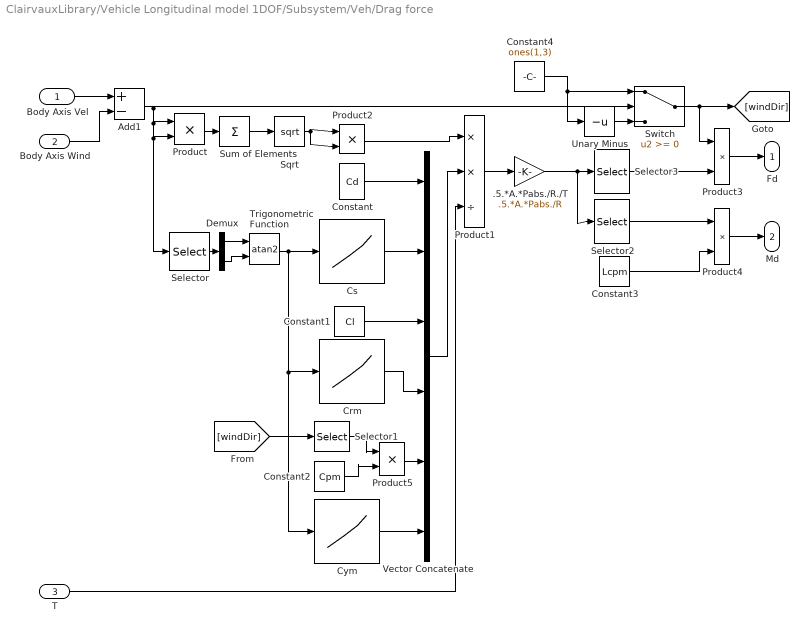
== system ClairvauxLibrary/Vehicle Longitudinal model 1DOF/Subsystem/Veh/Drag force ==
  Body Axis Vel : Inport
  Body Axis Wind : Inport  Port=2
  T : Inport  Port=3  OutMin=1
  .5.*A.*Pabs./R./T : Gain  Gain=.5.*A.*Pabs./R
  Add1 : Sum  Inputs=+-
  Constant : Constant  Value=Cd
  Constant1 : Constant  Value=Cl
  Constant2 : Constant  Value=Cpm
  Constant3 : Constant  Value=Lcpm
  Constant4 : Constant  Value=ones(1,3)
  Crm : Lookup_n-D  NumberOfTableDimensions=1  BreakpointsForDimension1=[-1 1]  Table=[0 0]  InternalRulePriority=Speed  RndMeth=Simplest  InputSameDT=on
  Cs : Lookup_n-D  NumberOfTableDimensions=1  BreakpointsForDimension1=beta_w  Table=Cs  ExtrapMethod=Clip  InternalRulePriority=Speed  RndMeth=Simplest  InputSameDT=on
  Cym : Lookup_n-D  NumberOfTableDimensions=1  BreakpointsForDimension1=beta_w  Table=Cym  InternalRulePriority=Speed  RndMeth=Simplest  InputSameDT=on
  Demux : Demux  Outputs=2
  Product{,2..5} (5 alike) : Product
  Product1 : Product  Inputs=**/
  Selector : Selector  InputPortWidth=3  IndexOptions=Index vector (dialog)  Indices=[2 1]  OutputSizes=1
  Selector1 : Selector  InputPortWidth=3  IndexOptions=Index vector (dialog)  Indices=[1]  OutputSizes=1
  Selector2 : Selector  InputPortWidth=6  IndexOptions=Index vector (dialog)  Indices=[4:6]  OutputSizes=1
  Selector3 : Selector  InputPortWidth=6  IndexOptions=Index vector (dialog)  Indices=[1:3]  OutputSizes=1
  Sqrt : Sqrt  SaturateOnIntegerOverflow=on
  Sum of Elements : Sum  Inputs=+
  Switch : Switch  ZeroCross=off
  Trigonometric Function : Trigonometry  Operator=atan2  OutputSignalType=real
  Unary Minus : UnaryMinus
  Vector Concatenate : Concatenate  NumInputs=6
  Fd : Outport  VectorParamsAs1DForOutWhenUnconnected=off
  Md : Outport  Port=2  VectorParamsAs1DForOutWhenUnconnected=off
  wires:
  Selector1/1 -> Product5/1
  T/1 -> Product1/3
  Demux/1 -> Trigonometric Function/1
  Constant4/1 -> Unary Minus/1, Switch/1
  Constant2/1 -> Product5/2
  Vector Concatenate/1 -> Product1/2
  [windDir] -> Selector1/1
  Switch/1 -> [windDir], Product3/1
  Constant3/1 -> Product4/2
  Crm/1 -> Vector Concatenate/4
  Unary Minus/1 -> Switch/3
  Body Axis Wind/1 -> Add1/2
  Selector3/1 -> Product3/2
  Cym/1 -> Vector Concatenate/6
  Selector2/1 -> Product4/1
  Product5/1 -> Vector Concatenate/5
  Constant1/1 -> Vector Concatenate/3
  Product4/1 -> Md/1
  Product/1 -> Sum of Elements/1
  Product2/1 -> Product1/1
  Selector/1 -> Demux/1
  Product1/1 -> .5.*A.*Pabs./R./T/1
  Trigonometric Function/1 -> Cs/1, Crm/1, Cym/1
  Body Axis Vel/1 -> Add1/1
  Add1/1 -> Switch/2, Selector/1, Product/2, Product/1
  Demux/2 -> Trigonometric Function/2
  Product3/1 -> Fd/1
  Constant/1 -> Vector Concatenate/1
  Cs/1 -> Vector Concatenate/2
  .5.*A.*Pabs./R./T/1 -> Selector3/1, Selector2/1
  Sqrt/1 -> Product2/1, Product2/2
  Sum of Elements/1 -> Sqrt/1

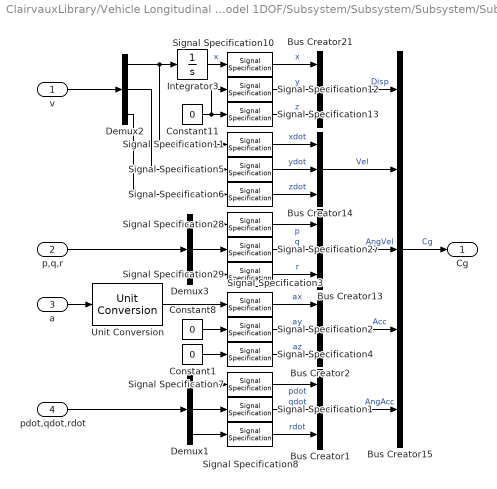
== system ClairvauxLibrary/Vehicle Longitudinal model 1DOF/Subsystem/Subsystem/Subsystem/Subsystem ==
  v : Inport
  p,q,r : Inport  Port=2
  a : Inport  Port=3
  pdot,qdot,rdot : Inport  Port=4
  Bus Creator{1..2,13..14,21} (5 alike) : BusCreator  Inputs=3
  Bus Creator15 : BusCreator  Inputs=5
  Constant1 : Constant  Value=0
  Constant11 : Constant  Value=0
  Constant8 : Constant  Value=0
  Demux1 : Demux  Outputs=3
  Demux2 : Demux  Outputs=3
  Demux3 : Demux  Outputs=3
  Integrator3 : Integrator  InitialCondition=xdot_o
  Signal Specification1 : SignalSpecification  Unit=rad/s^2
  Signal Specification10 : SignalSpecification  Unit=m
  Signal Specification11 : SignalSpecification  Unit=m/s
  Signal Specification12 : SignalSpecification  Unit=m
  Signal Specification13 : SignalSpecification  Unit=m
  Signal Specification2 : SignalSpecification  Unit=gn
  Signal Specification27 : SignalSpecification  Unit=rad/s
  Signal Specification28 : SignalSpecification  Unit=rad/s
  Signal Specification29 : SignalSpecification  Unit=rad/s
  Signal Specification3 : SignalSpecification  Unit=gn
  Signal Specification4 : SignalSpecification  Unit=gn
  Signal Specification5 : SignalSpecification  Unit=m/s
  Signal Specification6 : SignalSpecification  Unit=m/s
  Signal Specification7 : SignalSpecification  Unit=rad/s^2
  Signal Specification8 : SignalSpecification  Unit=rad/s^2
  Unit Conversion : UnitConversion
  Cg : Outport  VectorParamsAs1DForOutWhenUnconnected=off
  wires:
  a/1 -> Unit Conversion/1
  Signal Specification3/1 -> Bus Creator2/1  "ax"
  Bus Creator21/1 -> Bus Creator15/1  "Disp"
  Bus Creator14/1 -> Bus Creator15/2  "Vel"
  Demux2/2 -> Signal Specification5/1
  v/1 -> Demux2/1
  Signal Specification12/1 -> Bus Creator21/2  "y"
  Signal Specification5/1 -> Bus Creator14/2  "ydot"
  Demux2/3 -> Signal Specification6/1
  Signal Specification6/1 -> Bus Creator14/3  "zdot"
  Demux3/3 -> Signal Specification29/1
  Signal Specification11/1 -> Bus Creator14/1  "xdot"
  Signal Specification2/1 -> Bus Creator2/2  "ay"
  Signal Specification29/1 -> Bus Creator13/3  "r"
  pdot,qdot,rdot/1 -> Demux1/1
  Bus Creator15/1 -> Cg/1  "Cg"
  Signal Specification13/1 -> Bus Creator21/3  "z"
  Signal Specification28/1 -> Bus Creator13/1  "p"
  Demux2/1 -> Integrator3/1, Signal Specification11/1
  Bus Creator13/1 -> Bus Creator15/3  "AngVel"
  Signal Specification4/1 -> Bus Creator2/3  "az"
  Constant8/1 -> Signal Specification2/1
  Constant1/1 -> Signal Specification4/1
  Constant11/1 -> Signal Specification13/1, Signal Specification12/1
  Signal Specification10/1 -> Bus Creator21/1  "x"
  Signal Specification1/1 -> Bus Creator1/2  "qdot"
  Demux3/2 -> Signal Specification27/1
  Demux1/2 -> Signal Specification1/1
  Integrator3/1 -> Signal Specification10/1  "x"
  Signal Specification7/1 -> Bus Creator1/1  "pdot"
  Demux3/1 -> Signal Specification28/1
  Demux1/1 -> Signal Specification7/1
  Bus Creator2/1 -> Bus Creator15/4  "Acc"
  Signal Specification8/1 -> Bus Creator1/3  "rdot"
  Demux1/3 -> Signal Specification8/1
  Signal Specification27/1 -> Bus Creator13/2  "q"
  p,q,r/1 -> Demux3/1
  Bus Creator1/1 -> Bus Creator15/5  "AngAcc"
  Unit Conversion/1 -> Signal Specification3/1

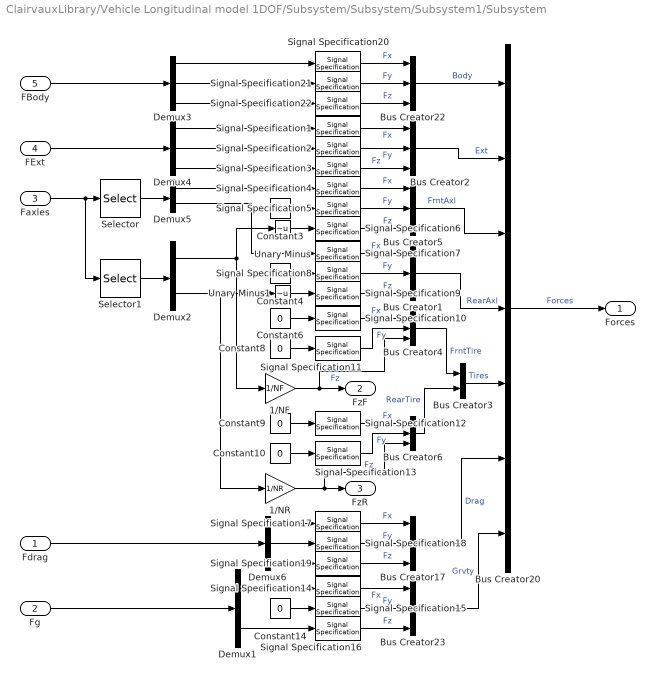
== system ClairvauxLibrary/Vehicle Longitudinal model 1DOF/Subsystem/Subsystem/Subsystem1/Subsystem ==
  Fdrag : Inport
  Fg : Inport  Port=2
  Faxles : Inport  Port=3
  FExt : Inport  Port=4
  FBody : Inport  Port=5
  1/NF : Gain  Gain=1/NF
  1/NR : Gain  Gain=1/NR
  Bus Creator{1..2,4..6,17,22..23} (8 alike) : BusCreator  Inputs=3
  Bus Creator20 : BusCreator  Inputs=7
  Bus Creator3 : BusCreator  Inputs=2
  Constant{3..4,6,8..10,14} (7 alike) : Constant  Value=0
  Demux1 : Demux  Outputs=2
  Demux2 : Demux  Outputs=2
  Demux3 : Demux  Outputs=3
  Demux4 : Demux  Outputs=3
  Demux5 : Demux  Outputs=2
  Demux6 : Demux  Outputs=3
  Selector : Selector  NumberOfDimensions=2  InputPortWidth=3  IndexOptions=Select all,Index vector (dialog)  Indices=[1],1  OutputSizes=1,1
  Selector1 : Selector  NumberOfDimensions=2  InputPortWidth=3  IndexOptions=Select all,Index vector (dialog)  Indices=[2],2  OutputSizes=1,1
  Signal Specification{1..22} (22 alike) : SignalSpecification  Unit=N
  Unary Minus : UnaryMinus
  Unary Minus1 : UnaryMinus
  Forces : Outport  VectorParamsAs1DForOutWhenUnconnected=off
  FzF : Outport  Port=2  VectorParamsAs1DForOutWhenUnconnected=off
  FzR : Outport  Port=3  VectorParamsAs1DForOutWhenUnconnected=off
  wires:
  Constant6/1 -> Signal Specification10/1
  Demux4/2 -> Signal Specification2/1
  Signal Specification7/1 -> Bus Creator1/1  "Fx"
  Signal Specification6/1 -> Bus Creator5/3  "Fz"
  Constant3/1 -> Signal Specification5/1
  Constant4/1 -> Signal Specification8/1
  Demux4/1 -> Signal Specification1/1
  Unary Minus1/1 -> Signal Specification9/1
  Constant8/1 -> Signal Specification11/1
  Constant10/1 -> Signal Specification13/1
  1/NR/1 -> FzR/1, Bus Creator6/3  "Fz"
  Selector/1 -> Demux5/1
  Signal Specification12/1 -> Bus Creator6/1  "Fx"
  Demux5/1 -> Signal Specification4/1
  Demux3/1 -> Signal Specification20/1
  Bus Creator3/1 -> Bus Creator20/5  "Tires"
  Fdrag/1 -> Demux6/1
  Faxles/1 -> Selector/1, Selector1/1
  Bus Creator1/1 -> Bus Creator20/4  "RearAxl"
  Bus Creator22/1 -> Bus Creator20/1  "Body"
  Signal Specification11/1 -> Bus Creator4/2  "Fy"
  Signal Specification20/1 -> Bus Creator22/1  "Fx"
  Signal Specification4/1 -> Bus Creator5/1  "Fx"
  Demux6/2 -> Signal Specification18/1
  Constant9/1 -> Signal Specification12/1
  Signal Specification5/1 -> Bus Creator5/2  "Fy"
  Signal Specification1/1 -> Bus Creator2/1  "Fx"
  Bus Creator5/1 -> Bus Creator20/3  "FrntAxl"
  Bus Creator23/1 -> Bus Creator20/7  "Grvty"
  Selector1/1 -> Demux2/1
  Signal Specification2/1 -> Bus Creator2/2  "Fy"
  Demux6/1 -> Signal Specification17/1
  Signal Specification22/1 -> Bus Creator22/3  "Fz"
  Signal Specification15/1 -> Bus Creator23/2  "Fy"
  Signal Specification3/1 -> Bus Creator2/3  "Fz"
  Signal Specification13/1 -> Bus Creator6/2  "Fy"
  Demux6/3 -> Signal Specification19/1
  Demux2/1 -> Unary Minus/1, 1/NF/1
  1/NF/1 -> FzF/1, Bus Creator4/3  "Fz"
  Signal Specification9/1 -> Bus Creator1/3  "Fz"
  Signal Specification14/1 -> Bus Creator23/1  "Fx"
  FBody/1 -> Demux3/1
  Bus Creator20/1 -> Forces/1  "Forces"
  Demux1/1 -> Signal Specification14/1
  Signal Specification18/1 -> Bus Creator17/2  "Fy"
  Bus Creator2/1 -> Bus Creator20/2  "Ext"
  Demux4/3 -> Signal Specification3/1
  Unary Minus/1 -> Signal Specification6/1
  Demux5/2 -> Signal Specification7/1
  Bus Creator4/1 -> Bus Creator3/1  "FrntTire"
  Signal Specification10/1 -> Bus Creator4/1  "Fx"
  Demux3/2 -> Signal Specification21/1
  Constant14/1 -> Signal Specification15/1
  Signal Specification17/1 -> Bus Creator17/1  "Fx"
  Signal Specification21/1 -> Bus Creator22/2  "Fy"
  Bus Creator17/1 -> Bus Creator20/6  "Drag"
  Demux2/2 -> Unary Minus1/1, 1/NR/1
  Bus Creator6/1 -> Bus Creator3/2  "RearTire"
  Signal Specification19/1 -> Bus Creator17/3  "Fz"
  Demux1/2 -> Signal Specification16/1
  Signal Specification8/1 -> Bus Creator1/2  "Fy"
  Signal Specification16/1 -> Bus Creator23/3  "Fz"
  Fg/1 -> Demux1/1
  FExt/1 -> Demux4/1
  Demux3/3 -> Signal Specification22/1

== system ClairvauxLibrary/Vehicle Longitudinal model 1DOF/Subsystem/Subsystem/Subsystem3/Subsystem ==
  U,w : Inport
  Theta : Inport  Port=2
  Constant : Constant  Value=0
  Mux3 : Mux  Inputs=3
  Mux4 : Mux  Inputs=3
  Product : Product  Multiplication=Matrix(*)  SaturateOnIntegerOverflow=on  OutDataTypeStr=Inherit: Same as first input
  Rotation Angles to Direction Cosine Matrix : sharedtransform/Rotation Angles to Direction Cosine Matrix  rotationOrder=ZYX  aMode=aMode
      settings: SourceProductBaseCode=AE,PW,MT,UV,VE,VP
  Selector : Selector  InputPortWidth=2  IndexOptions=Index vector (dialog)  Indices=1  OutputSizes=1
  Selector1 : Selector  InputPortWidth=3  IndexOptions=Index vector (dialog)  Indices=[1 3]  OutputSizes=1
  Selector2 : Selector  InputPortWidth=2  IndexOptions=Index vector (dialog)  Indices=2  OutputSizes=1
  Transpose : Math  Operator=transpose  SignedPower=on  SaturateOnIntegerOverflow=on
  Ue,we : Outport  Unit=m/s  VectorParamsAs1DForOutWhenUnconnected=off
  wires:
  Mux4/1 -> Product/2
  Mux3/1 -> Rotation Angles to Direction Cosine Matrix/1
  Transpose/1 -> Product/1
  Theta/1 -> Mux3/2
  U,w/1 -> Selector2/1, Selector/1
  Selector2/1 -> Mux4/3
  Rotation Angles to Direction Cosine Matrix/1 -> Transpose/1
  Selector1/1 -> Ue,we/1
  Product/1 -> Selector1/1
  Selector/1 -> Mux4/1
  Constant/1 -> Mux3/3, Mux4/2, Mux3/1

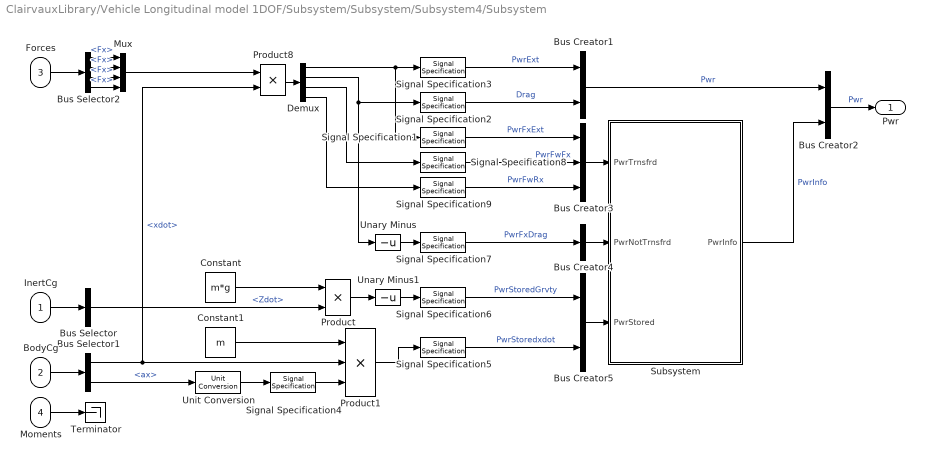
== system ClairvauxLibrary/Vehicle Longitudinal model 1DOF/Subsystem/Subsystem/Subsystem4/Subsystem ==
  InertCg : Inport
  BodyCg : Inport  Port=2
  Forces : Inport  Port=3
  Moments : Inport  Port=4
  Bus Creator1 : BusCreator  Inputs=2
  Bus Creator2 : BusCreator  Inputs=2
  Bus Creator3 : BusCreator  Inputs=3
  Bus Creator4 : BusCreator  Inputs=1
  Bus Creator5 : BusCreator  Inputs=2
  Bus Selector : BusSelector  OutputSignals=Cg.Vel.Zdot
  Bus Selector1 : BusSelector  OutputSignals=Cg.Vel.xdot,Cg.Acc.ax
  Bus Selector2 : BusSelector  OutputSignals=Ext.Fx,Drag.Fx,FrntAxl.Fx,RearAxl.Fx
  Constant : Constant  Value=m*g
  Constant1 : Constant  Value=m
  Demux : Demux
  Mux : Mux
  Product : Product
  Product1 : Product  Inputs=3
  Product8 : Product
  Signal Specification{1..3,5..9} (8 alike) : SignalSpecification  Unit=W
  Signal Specification4 : SignalSpecification  Unit=m/s^2
  Subsystem : Subsystem
  Terminator : Terminator
  Unary Minus : UnaryMinus
  Unary Minus1 : UnaryMinus
  Unit Conversion : UnitConversion
  Pwr : Outport  VectorParamsAs1DForOutWhenUnconnected=off
  wires:
  Signal Specification1/1 -> Bus Creator3/1  "PwrFxExt"
  Bus Selector2/2 -> Mux/2  "<Fx>"
  InertCg/1 -> Bus Selector/1
  Signal Specification3/1 -> Bus Creator1/1  "PwrExt"
  Bus Creator2/1 -> Pwr/1  "Pwr"
  Bus Selector2/4 -> Mux/4  "<Fx>"
  Product8/1 -> Demux/1
  Forces/1 -> Bus Selector2/1
  Moments/1 -> Terminator/1
  Demux/3 -> Signal Specification8/1
  Bus Creator5/1 -> Subsystem/3(PwrStored)
  Unary Minus/1 -> Signal Specification7/1
  Bus Selector1/2 -> Unit Conversion/1  "<ax>"
  Product1/1 -> Signal Specification5/1
  BodyCg/1 -> Bus Selector1/1
  Signal Specification4/1 -> Product1/3
  Unary Minus1/1 -> Signal Specification6/1
  Mux/1 -> Product8/1
  Constant1/1 -> Product1/1
  Bus Selector2/3 -> Mux/3  "<Fx>"
  Bus Creator1/1 -> Bus Creator2/1  "Pwr"
  Product/1 -> Unary Minus1/1
  Bus Creator4/1 -> Subsystem/2(PwrNotTrnsfrd)
  Unit Conversion/1 -> Signal Specification4/1
  Bus Selector2/1 -> Mux/1  "<Fx>"
  Demux/2 -> Unary Minus/1, Signal Specification2/1
  Bus Creator3/1 -> Subsystem/1(PwrTrnsfrd)
  Bus Selector1/1 -> Product8/2, Product1/2  "<xdot>"
  Constant/1 -> Product/1
  Signal Specification7/1 -> Bus Creator4/1  "PwrFxDrag"
  Subsystem/1(PwrInfo) -> Bus Creator2/2  "PwrInfo"
  Demux/1 -> Signal Specification3/1, Signal Specification1/1
  Signal Specification6/1 -> Bus Creator5/1  "PwrStoredGrvty"
  Signal Specification5/1 -> Bus Creator5/2  "PwrStoredxdot"
  Bus Selector/1 -> Product/2  "<Zdot>"
  Demux/4 -> Signal Specification9/1
  Signal Specification9/1 -> Bus Creator3/3  "PwrFwRx"
  Signal Specification8/1 -> Bus Creator3/2  "PwrFwFx"
  Signal Specification2/1 -> Bus Creator1/2  "Drag"

== system ClairvauxLibrary/Vehicle Longitudinal model 1DOF/Subsystem/Subsystem/Subsystem5/Subsystem ==
  InertCg : Inport
  BdyFrmCg : Inport  Port=2
  Forces : Inport  Port=3
  Power : Inport  Port=4
  Moments : Inport  Port=5
  WhlAngF : Inport  Port=6
  WhlAngR : Inport  Port=7
  Bus Creator1 : BusCreator  Inputs=6
  Bus Creator2 : BusCreator  Inputs=3
  Bus Creator3 : BusCreator  Inputs=2
  Bus Creator4 : BusCreator  Inputs=2
  Bus Selector : BusSelector  OutputSignals=Pwr,PwrInfo
  Demux : Demux  Outputs=2
  Demux1 : Demux  Outputs=2
  Subsystem : Subsystem  mask{R_T1=a, R_T2=0, R_T3=h}
      mask prompts: R_T1 "x position from CG to suspension hardpoint:"; R_T2 "y position from CG to suspension hardpoint:"; R_T3 "z position from CG to suspension hardpoint:"
  Subsystem1 : $bdroot/Vehicle Longitudinal model 1DOF/Subsystem/Subsystem/Subsystem5/Subsystem/Subsystem  R_T1=-b  R_T2=0  R_T3=h
  InertFrm : Outport  VectorParamsAs1DForOutWhenUnconnected=off
  BdyFrm : Outport  Port=2  VectorParamsAs1DForOutWhenUnconnected=off
  PwrInfo : Outport  Port=3  VectorParamsAs1DForOutWhenUnconnected=off
  wires:
  Demux1/1 -> Bus Creator4/1  "WhlAngRL"
  Power/1 -> Bus Selector/1  "Pwr"
  Demux/2 -> Bus Creator3/2  "WhlAngFR"
  Bus Creator4/1 -> Subsystem1/3  "Steer"
  Bus Selector/1 -> Bus Creator1/6  "<Pwr>"
  Demux1/2 -> Bus Creator4/2  "WhlAngRR"
  Demux/1 -> Bus Creator3/1  "WhlAngFL"
  WhlAngR/1 -> Demux1/1  "WhlAngR"
  Bus Selector/2 -> PwrInfo/1  "<PwrInfo>"
  WhlAngF/1 -> Demux/1  "WhlAngF"
  InertCg/1 -> Subsystem1/1, Subsystem/1(InertFrmCg), Bus Creator2/1  "Cg"
  Moments/1 -> Bus Creator1/3  "Moments"
  Forces/1 -> Bus Creator1/2  "Forces"
  Subsystem1/1 -> Bus Creator2/3  "RearAxl"
  Subsystem/1(Inertial) -> Bus Creator2/2  "FrntAxl"
  Bus Creator1/1 -> BdyFrm/1  "BdyFrm"
  Bus Creator2/1 -> InertFrm/1  "InertFrm"
  Bus Creator3/1 -> Subsystem/3(Steer)  "Steer"
  BdyFrmCg/1 -> Bus Creator1/1, Subsystem1/2, Subsystem/2(BdyFrmCg)  "Cg"
  Subsystem/2(Body) -> Bus Creator1/4  "FrntAxl"
  Subsystem1/2 -> Bus Creator1/5  "RearAxl"

== system ClairvauxLibrary/Vehicle Longitudinal model 1DOF/Subsystem/Subsystem/Subsystem4/Subsystem/Subsystem ==
  PwrTrnsfrd : Inport
  PwrNotTrnsfrd : Inport  Port=2
  PwrStored : Inport  Port=3
  Bus Creator : BusCreator  Inputs=3
  Signal Specification : SignalSpecification  Unit=W
  PwrInfo : Outport  VectorParamsAs1DForOutWhenUnconnected=off
  wires:
  PwrNotTrnsfrd/1 -> Bus Creator/2  "PwrNotTrnsfrd"
  PwrStored/1 -> Bus Creator/3  "PwrStored"
  PwrTrnsfrd/1 -> Bus Creator/1  "PwrTrnsfrd"
  Bus Creator/1 -> Signal Specification/1
  Signal Specification/1 -> PwrInfo/1  "PwrInfo"
